simulink subsystem "BMS"  (R2024b)
settings: Solver=VariableStepAuto  StartTime=0.0  StopTime=10.0  RelTol=1e-3
undefined symbols (not defined in the file): Ambient, battery_builder_rtmsupport, ChargeKp, ChargerCC_A, ChargerKi, CoolantTemp, CurrOffset, gcbh, MaxChrgCurLim, MaxDchrgCurLim, MaxThLmt, MaxVoltLmt, MinThLmt, MinVoltLmt, Np, VoltOffset
libraries: nesl_utility x27, Batteries_lib x20, fl_lib x11, BatteryThermalManagement x1, BatteryCurrentManagement x1, BatteryBalancing x1
(part 2 of 4)

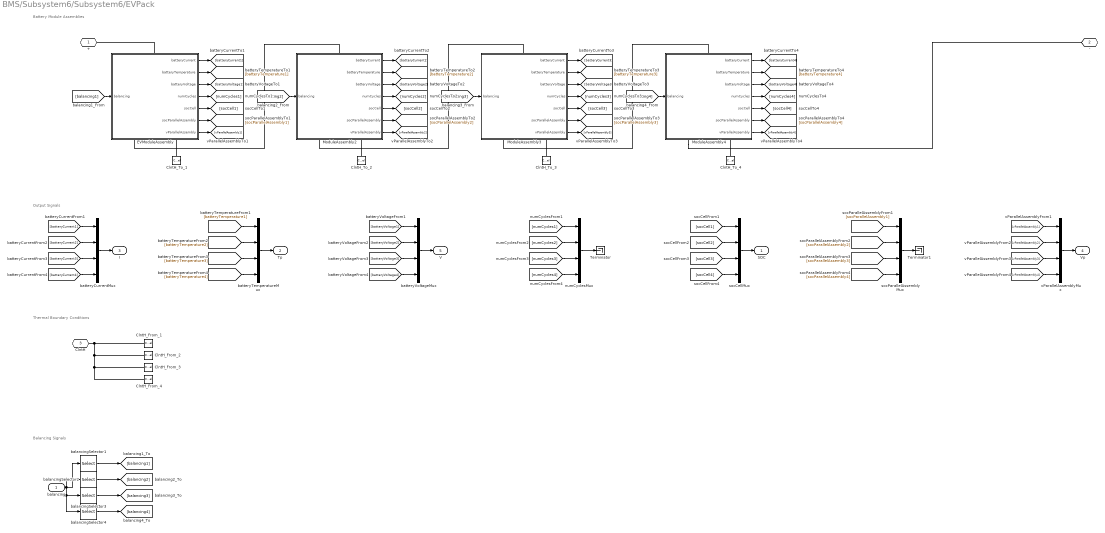
== system BMS/Subsystem6/Subsystem6/EVPack ==
  note: Balancing Signals
  note: Thermal Boundary Conditions
  note: Output Signals
  note: Battery Module Assemblies
  balancing : Inport  PortDimensions=100
  ClntH_From_1 : ConnectionLabel  Label=clntH_1
  ClntH_From_2 : ConnectionLabel  Label=clntH_2
  ClntH_From_3 : ConnectionLabel  Label=clntH_3
  ClntH_From_4 : ConnectionLabel  Label=clntH_4
  ClntH_To_1 : ConnectionLabel  Label=clntH_1
  ClntH_To_2 : ConnectionLabel  Label=clntH_2
  ClntH_To_3 : ConnectionLabel  Label=clntH_3
  ClntH_To_4 : ConnectionLabel  Label=clntH_4
  EVModuleAssembly : Subsystem  LoadFcn=battery_builder_rtmsupport('loadfcn',gcbh);
      settings: CopyFcn=battery_builder_rtmsupport('copyfcn',gcbh);  PreCopyFcn=battery_builder_rtmsupport('precopyfcn',gcbh);  PreDeleteFcn=battery_builder_rtmsupport('predeletefcn',gcbh);  PortSchema="{\"entries\":[{\"content\":{\"sides\":[{\"content\":{\"connectorIds\":[\"LConn1\"]},\"type\":\"ConnectorPlacement.EquallySpacedRectSide\",\"uuid\":\"3fa46d70-8935-4e0c-abb4-9c9b0d92b81b\"},{\"content\":{\"connectorIds\":[\"RConn1\",\"RConn2\"],\"side\":\"RIGHT\"},\"type\":\"ConnectorPlacement.EquallySpacedRectSide\",\"uuid\":\"6c8ace96-c3fc-41f9-a773-88712ff4ff02\"},{\"content\":{\"connectorIds\":[\"In1\"],\"side\":\"TOP\"},\"type\":\"ConnectorPlacement.EquallySpacedRectSide\",\"uuid\":\"16b2d02e-c4ca-4b99-b91f-f3cca8ade205\"},{\"content\":{\"connectorIds\":[\"Out1\",\"Out2\",\"Out3\",\"Out4\",\"Out5\",\"Out6\",\"Out7\"],\"side\":\"BOTTOM\"},\"type\":\"ConnectorPlacement.EquallySpacedRectSide\",\"uuid\":\"90084359-4b5d-48c4-95f3-9d483f7e7445\"}]},\"type\":\"ConnectorPlacement.EquallySpacedConnector\",\"uuid\":\"91dc49f4-abd8-4582-9e7e-23b88d2919e3\"}],\"packageUris\":[\"http://schema.mathworks.com/mf0/Connector/R2020b\"],\"version\":\"1.0\"}"
      mask Display: image('$imagefile')
  ModuleAssembly2 : Subsystem  LoadFcn=battery_builder_rtmsupport('loadfcn',gcbh);
      settings: CopyFcn=battery_builder_rtmsupport('copyfcn',gcbh);  PreCopyFcn=battery_builder_rtmsupport('precopyfcn',gcbh);  PreDeleteFcn=battery_builder_rtmsupport('predeletefcn',gcbh);  PortSchema="{\"entries\":[{\"content\":{\"sides\":[{\"content\":{\"connectorIds\":[\"LConn1\"]},\"type\":\"ConnectorPlacement.EquallySpacedRectSide\",\"uuid\":\"3fa46d70-8935-4e0c-abb4-9c9b0d92b81b\"},{\"content\":{\"connectorIds\":[\"RConn1\",\"RConn2\"],\"side\":\"RIGHT\"},\"type\":\"ConnectorPlacement.EquallySpacedRectSide\",\"uuid\":\"6c8ace96-c3fc-41f9-a773-88712ff4ff02\"},{\"content\":{\"connectorIds\":[\"In1\"],\"side\":\"TOP\"},\"type\":\"ConnectorPlacement.EquallySpacedRectSide\",\"uuid\":\"16b2d02e-c4ca-4b99-b91f-f3cca8ade205\"},{\"content\":{\"connectorIds\":[\"Out1\",\"Out2\",\"Out3\",\"Out4\",\"Out5\",\"Out6\",\"Out7\"],\"side\":\"BOTTOM\"},\"type\":\"ConnectorPlacement.EquallySpacedRectSide\",\"uuid\":\"90084359-4b5d-48c4-95f3-9d483f7e7445\"}]},\"type\":\"ConnectorPlacement.EquallySpacedConnector\",\"uuid\":\"91dc49f4-abd8-4582-9e7e-23b88d2919e3\"}],\"packageUris\":[\"http://schema.mathworks.com/mf0/Connector/R2020b\"],\"version\":\"1.0\"}"
      mask Display: image('$imagefile')
  ModuleAssembly3 : Subsystem  LoadFcn=battery_builder_rtmsupport('loadfcn',gcbh);
      settings: CopyFcn=battery_builder_rtmsupport('copyfcn',gcbh);  PreCopyFcn=battery_builder_rtmsupport('precopyfcn',gcbh);  PreDeleteFcn=battery_builder_rtmsupport('predeletefcn',gcbh);  PortSchema="{\"entries\":[{\"content\":{\"sides\":[{\"content\":{\"connectorIds\":[\"LConn1\"]},\"type\":\"ConnectorPlacement.EquallySpacedRectSide\",\"uuid\":\"3fa46d70-8935-4e0c-abb4-9c9b0d92b81b\"},{\"content\":{\"connectorIds\":[\"RConn1\",\"RConn2\"],\"side\":\"RIGHT\"},\"type\":\"ConnectorPlacement.EquallySpacedRectSide\",\"uuid\":\"6c8ace96-c3fc-41f9-a773-88712ff4ff02\"},{\"content\":{\"connectorIds\":[\"In1\"],\"side\":\"TOP\"},\"type\":\"ConnectorPlacement.EquallySpacedRectSide\",\"uuid\":\"16b2d02e-c4ca-4b99-b91f-f3cca8ade205\"},{\"content\":{\"connectorIds\":[\"Out1\",\"Out2\",\"Out3\",\"Out4\",\"Out5\",\"Out6\",\"Out7\"],\"side\":\"BOTTOM\"},\"type\":\"ConnectorPlacement.EquallySpacedRectSide\",\"uuid\":\"90084359-4b5d-48c4-95f3-9d483f7e7445\"}]},\"type\":\"ConnectorPlacement.EquallySpacedConnector\",\"uuid\":\"91dc49f4-abd8-4582-9e7e-23b88d2919e3\"}],\"packageUris\":[\"http://schema.mathworks.com/mf0/Connector/R2020b\"],\"version\":\"1.0\"}"
      mask Display: image('$imagefile')
  ModuleAssembly4 : Subsystem  LoadFcn=battery_builder_rtmsupport('loadfcn',gcbh);
      settings: CopyFcn=battery_builder_rtmsupport('copyfcn',gcbh);  PreCopyFcn=battery_builder_rtmsupport('precopyfcn',gcbh);  PreDeleteFcn=battery_builder_rtmsupport('predeletefcn',gcbh);  PortSchema="{\"entries\":[{\"content\":{\"sides\":[{\"content\":{\"connectorIds\":[\"LConn1\"]},\"type\":\"ConnectorPlacement.EquallySpacedRectSide\",\"uuid\":\"3fa46d70-8935-4e0c-abb4-9c9b0d92b81b\"},{\"content\":{\"connectorIds\":[\"RConn1\",\"RConn2\"],\"side\":\"RIGHT\"},\"type\":\"ConnectorPlacement.EquallySpacedRectSide\",\"uuid\":\"6c8ace96-c3fc-41f9-a773-88712ff4ff02\"},{\"content\":{\"connectorIds\":[\"In1\"],\"side\":\"TOP\"},\"type\":\"ConnectorPlacement.EquallySpacedRectSide\",\"uuid\":\"16b2d02e-c4ca-4b99-b91f-f3cca8ade205\"},{\"content\":{\"connectorIds\":[\"Out1\",\"Out2\",\"Out3\",\"Out4\",\"Out5\",\"Out6\",\"Out7\"],\"side\":\"BOTTOM\"},\"type\":\"ConnectorPlacement.EquallySpacedRectSide\",\"uuid\":\"90084359-4b5d-48c4-95f3-9d483f7e7445\"}]},\"type\":\"ConnectorPlacement.EquallySpacedConnector\",\"uuid\":\"91dc49f4-abd8-4582-9e7e-23b88d2919e3\"}],\"packageUris\":[\"http://schema.mathworks.com/mf0/Connector/R2020b\"],\"version\":\"1.0\"}"
      mask Display: image('$imagefile')
  Terminator : Terminator
  Terminator1 : Terminator
  balancingSelector1 : Selector  InputPortWidth=100  IndexOptions=Index vector (dialog)  Indices="[1   2   3   4   5   6   7   8   9  10  11  12  13  14  15  16  17  18  19  20  21  22  23  24  25]"  OutputSizes=1
  balancingSelector2 : Selector  InputPortWidth=100  IndexOptions=Index vector (dialog)  Indices="[26  27  28  29  30  31  32  33  34  35  36  37  38  39  40  41  42  43  44  45  46  47  48  49  50]"  OutputSizes=1
  balancingSelector3 : Selector  InputPortWidth=100  IndexOptions=Index vector (dialog)  Indices="[51  52  53  54  55  56  57  58  59  60  61  62  63  64  65  66  67  68  69  70  71  72  73  74  75]"  OutputSizes=1
  balancingSelector4 : Selector  InputPortWidth=100  IndexOptions=Index vector (dialog)  Indices="[76   77   78   79   80   81   82   83   84   85   86   87   88   89   90   91   92   93   94   95   96   97   98   99  100]"  OutputSizes=1
  batteryCurrentMux : Mux
  batteryTemperatureMux : Mux
  batteryVoltageMux : Mux
  numCyclesMux : Mux
  socCellMux : Mux
  socParallelAssemblyMux : Mux
  vParallelAssemblyMux : Mux
  + : PMIOPort  Side=Left
  - : PMIOPort  Port=2  Side=Right
  ClntH : PMIOPort  Port=3  Side=Right  ConnectionType=Connection: foundation.thermal.thermal
  SOC : Outport
  Tp : Outport  Port=2
  I : Outport  Port=3
  Vp : Outport  Port=4
  V : Outport  Port=5
  wires:
  balancingSelector4/1 -> [balancing4]
  [balancing4] -> ModuleAssembly4/1(balancing)
  balancingSelector3/1 -> [balancing3]
  [balancing3] -> ModuleAssembly3/1(balancing)
  balancingSelector2/1 -> [balancing2]
  [balancing2] -> ModuleAssembly2/1(balancing)
  balancingSelector1/1 -> [balancing1]
  balancing/1 -> balancingSelector4/1, balancingSelector3/1, balancingSelector2/1, balancingSelector1/1
  [balancing1] -> EVModuleAssembly/1(balancing)
  [vParallelAssembly4] -> vParallelAssemblyMux/4
  ModuleAssembly4/7(vParallelAssembly) -> [vParallelAssembly4]
  [socParallelAssembly4] -> socParallelAssemblyMux/4
  ModuleAssembly4/6(socParallelAssembly) -> [socParallelAssembly4]
  [socCell4] -> socCellMux/4
  ModuleAssembly4/5(socCell) -> [socCell4]
  [numCycles4] -> numCyclesMux/4
  ModuleAssembly4/4(numCycles) -> [numCycles4]
  [batteryVoltage4] -> batteryVoltageMux/4
  ModuleAssembly4/3(batteryVoltage) -> [batteryVoltage4]
  [batteryTemperature4] -> batteryTemperatureMux/4
  ModuleAssembly4/2(batteryTemperature) -> [batteryTemperature4]
  [batteryCurrent4] -> batteryCurrentMux/4
  ModuleAssembly4/1(batteryCurrent) -> [batteryCurrent4]
  [vParallelAssembly3] -> vParallelAssemblyMux/3
  ModuleAssembly3/7(vParallelAssembly) -> [vParallelAssembly3]
  [socParallelAssembly3] -> socParallelAssemblyMux/3
  ModuleAssembly3/6(socParallelAssembly) -> [socParallelAssembly3]
  [socCell3] -> socCellMux/3
  ModuleAssembly3/5(socCell) -> [socCell3]
  [numCycles3] -> numCyclesMux/3
  ModuleAssembly3/4(numCycles) -> [numCycles3]
  [batteryVoltage3] -> batteryVoltageMux/3
  ModuleAssembly3/3(batteryVoltage) -> [batteryVoltage3]
  [batteryTemperature3] -> batteryTemperatureMux/3
  ModuleAssembly3/2(batteryTemperature) -> [batteryTemperature3]
  [batteryCurrent3] -> batteryCurrentMux/3
  ModuleAssembly3/1(batteryCurrent) -> [batteryCurrent3]
  [vParallelAssembly2] -> vParallelAssemblyMux/2
  ModuleAssembly2/7(vParallelAssembly) -> [vParallelAssembly2]
  [socParallelAssembly2] -> socParallelAssemblyMux/2
  ModuleAssembly2/6(socParallelAssembly) -> [socParallelAssembly2]
  [socCell2] -> socCellMux/2
  ModuleAssembly2/5(socCell) -> [socCell2]
  [numCycles2] -> numCyclesMux/2
  ModuleAssembly2/4(numCycles) -> [numCycles2]
  [batteryVoltage2] -> batteryVoltageMux/2
  ModuleAssembly2/3(batteryVoltage) -> [batteryVoltage2]
  [batteryTemperature2] -> batteryTemperatureMux/2
  ModuleAssembly2/2(batteryTemperature) -> [batteryTemperature2]
  [batteryCurrent2] -> batteryCurrentMux/2
  ModuleAssembly2/1(batteryCurrent) -> [batteryCurrent2]
  [vParallelAssembly1] -> vParallelAssemblyMux/1
  vParallelAssemblyMux/1 -> Vp/1
  EVModuleAssembly/7(vParallelAssembly) -> [vParallelAssembly1]
  [socParallelAssembly1] -> socParallelAssemblyMux/1
  socParallelAssemblyMux/1 -> Terminator1/1
  EVModuleAssembly/6(socParallelAssembly) -> [socParallelAssembly1]
  [socCell1] -> socCellMux/1
  socCellMux/1 -> SOC/1
  EVModuleAssembly/5(socCell) -> [socCell1]
  [numCycles1] -> numCyclesMux/1
  numCyclesMux/1 -> Terminator/1
  EVModuleAssembly/4(numCycles) -> [numCycles1]
  [batteryVoltage1] -> batteryVoltageMux/1
  batteryVoltageMux/1 -> V/1
  EVModuleAssembly/3(batteryVoltage) -> [batteryVoltage1]
  [batteryTemperature1] -> batteryTemperatureMux/1
  batteryTemperatureMux/1 -> Tp/1
  EVModuleAssembly/2(batteryTemperature) -> [batteryTemperature1]
  [batteryCurrent1] -> batteryCurrentMux/1
  batteryCurrentMux/1 -> I/1
  EVModuleAssembly/1(batteryCurrent) -> [batteryCurrent1]
  connections:
  ClntH_To_4/LConn1 -- ModuleAssembly4/RConn2
  ClntH_To_3/LConn1 -- ModuleAssembly3/RConn2
  ClntH_To_2/LConn1 -- ModuleAssembly2/RConn2
  ClntH_From_4/LConn1 -- ClntH/RConn1 -- ClntH_From_1/LConn1 -- ClntH_From_2/LConn1 -- ClntH_From_3/LConn1
  ClntH_To_1/LConn1 -- EVModuleAssembly/RConn2
  ModuleAssembly4/RConn1 -- -/RConn1
  EVModuleAssembly/LConn1 -- +/RConn1
  ModuleAssembly4/LConn1 -- ModuleAssembly3/RConn1
  ModuleAssembly3/LConn1 -- ModuleAssembly2/RConn1
  ModuleAssembly2/LConn1 -- EVModuleAssembly/RConn1

== system BMS/Subsystem6/BMS/Battery Protection Logic/State Flow ==
  Bus Element In11 : Inport  PortName=StateInput  Element=Current
  Bus Element In1 : Inport  PortName=StateInput  Element=CurLmt
  Bus Element In2 : Inport  PortName=StateInput  Element=Volt
  Bus Element In4 : Inport  PortName=StateInput  Element=Tp
  Bus Element In6 : Inport  PortName=StateInput  Element=BatSoC
  Bus Element In7 : Inport  PortName=StateInput  Element=BatCmd
  Bus Element In8 : Inport  PortName=StateInput  Element=FaultReset
  Bus Creator8 : BusCreator  Inputs=5
  Bus Creator9 : BusCreator  Inputs=4
  Delay{,1..3} (4 alike) : Delay  DelayLength=1
  Fault Protection : Stateflow chart  TreatAsAtomicUnit=on
      settings: PortSchema="{\"entries\":[{\"content\":{\"sides\":[{\"content\":{\"connectorIds\":[\"In1\",\"In2\",\"In3\",\"In4\",\"In5\",\"In6\",\"In7\"]},\"type\":\"ConnectorPlacement.EquallySpacedRectSide\",\"uuid\":\"7222f55a-2aef-4ca8-adbd-e86ed030f82f\"},{\"content\":{\"connectorIds\":[\"Out5\",\"Out6\",\"Out10\",\"Out9\",\"Out4\",\"Out1\",\"Out2\",\"Out3\",\"Out7\",\"Out8\"],\"side\":\"RIGHT\"},\"type\":\"ConnectorPlacement.EquallySpacedRectSide\",\"uuid\":\"bfa2f4e3-3563-4466-8725-57bf2336ec66\"},{\"content\":{\"connectorIds\":[],\"side\":\"TOP\"},\"type\":\"ConnectorPlacement.EquallySpacedRectSide\",\"uuid\":\"7b1e9a44-7135-4c45-bb2b-0152be29b46d\"}]},\"type\":\"ConnectorPlacement.EquallySpacedConnector\",\"uuid\":\"80032a24-3823-40c6-b797-ffbc29f7d345\"}],\"packageUris\":[\"http://schema.mathworks.com/mf0/Connector/R2020b\"],\"version\":\"1.0\"}"
  Out Bus Element : Outport  PortName=StateOut  Element=RelayRq
  Out Bus Element1 : Outport  PortName=StateOut  Element=BatSt
  Out Bus Element2 : Outport  PortName=StateOut  Element=Fault
  wires:
  Bus Element In7/1 -> Fault Protection/6(BatCmd)
  Bus Element In8/1 -> Fault Protection/7(FaultReset)
  Bus Element In2/1 -> Fault Protection/3(Volt)
  Bus Element In1/1 -> Fault Protection/2(CurLmt)
  Bus Element In11/1 -> Fault Protection/1(I)
  Bus Element In4/1 -> Fault Protection/4(Tp)
  Bus Element In6/1 -> Fault Protection/5(BatSoC)
  Bus Creator9/1 -> Out Bus Element/1  "RelayRq"
  Bus Creator8/1 -> Out Bus Element2/1  "Fault"
  Fault Protection/5(Rpos) -> Delay/1  "RelayPos"
  Fault Protection/6(Rneg) -> Delay1/1  "RelayNeg"
  Fault Protection/10(RelDchg) -> Delay2/1  "RelayDchg"
  Fault Protection/9(RelChg) -> Delay3/1  "RelayChg"
  Fault Protection/4(BatSt) -> Out Bus Element1/1  "BatSt"
  Fault Protection/2(FaultElec) -> Bus Creator8/2  "FaultElec"
  Fault Protection/3(FaultTh) -> Bus Creator8/3  "FaultTh"
  Fault Protection/7(FaultVolt) -> Bus Creator8/4  "FaultVolt"
  Fault Protection/8(FaultDisp) -> Bus Creator8/5  "FaultDisp"
  Fault Protection/1(FaultDet) -> Bus Creator8/1  "FaultDet"
  Delay/1 -> Bus Creator9/1  "RelayPos"
  Delay1/1 -> Bus Creator9/2  "RelayNeg"
  Delay2/1 -> Bus Creator9/3  "RelayDchg"
  Delay3/1 -> Bus Creator9/4  "RelayChg"

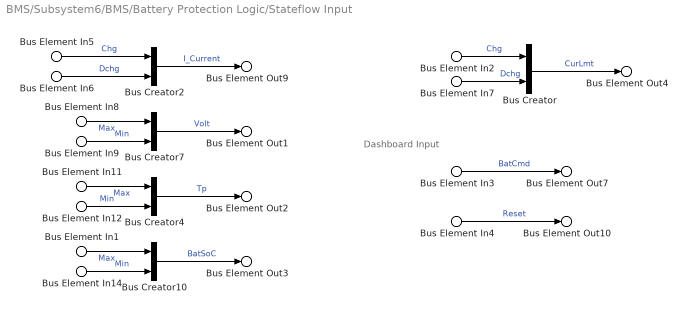
== system BMS/Subsystem6/BMS/Battery Protection Logic/Stateflow Input ==
  note: Dashboard Input
  Bus Element In1 : Inport  PortName=SoC  Element=CellSoCmax
  Bus Element In14 : Inport  PortName=SoC  Element=CellSoCmin
  Bus Element In2 : Inport  Port=2  PortName=Current  Element=CurChgLmt
  Bus Element In7 : Inport  Port=2  PortName=Current  Element=CurDchLmt
  Bus Element In5 : Inport  Port=2  PortName=Current  Element=CurChgDchg.Chg
  Bus Element In6 : Inport  Port=2  PortName=Current  Element=CurChgDchg.Dchg
  Bus Element In8 : Inport  Port=3  PortName=Sensor  Element=CellVoltMax
  Bus Element In9 : Inport  Port=3  PortName=Sensor  Element=CellVoltMin
  Bus Element In11 : Inport  Port=3  PortName=Sensor  Element=CellTempMax
  Bus Element In12 : Inport  Port=3  PortName=Sensor  Element=CellTempMin
  Bus Element In3 : Inport  Port=3  PortName=Sensor  Element=BatCmd
  Bus Element In4 : Inport  Port=3  PortName=Sensor  Element=Reset
  Bus Creator : BusCreator  Inputs=2  OutDataTypeStr=Bus: I_Current
  Bus Creator10 : BusCreator  Inputs=2  OutDataTypeStr=Bus: MaxMinLimit
  Bus Creator2 : BusCreator  Inputs=2  OutDataTypeStr=Bus: I_Current
  Bus Creator4 : BusCreator  Inputs=2  OutDataTypeStr=Bus: MaxMinLimit
  Bus Creator7 : BusCreator  Inputs=2  OutDataTypeStr=Bus: CellVoltage  NonVirtualBus=on
  Bus Element Out9 : Outport  PortName=StateInput  Element=Current
  Bus Element Out1 : Outport  PortName=StateInput  Element=Volt
  Bus Element Out2 : Outport  PortName=StateInput  Element=Tp
  Bus Element Out3 : Outport  PortName=StateInput  Element=BatSoC
  Bus Element Out4 : Outport  PortName=StateInput  Element=CurLmt
  Bus Element Out7 : Outport  PortName=StateInput  Element=BatCmd
  Bus Element Out10 : Outport  PortName=StateInput  Element=FaultReset
  wires:
  Bus Element In7/1 -> Bus Creator/2  "Dchg"
  Bus Element In2/1 -> Bus Creator/1  "Chg"
  Bus Creator7/1 -> Bus Element Out1/1  "Volt"
  Bus Creator2/1 -> Bus Element Out9/1  "I_Current"
  Bus Creator4/1 -> Bus Element Out2/1  "Tp"
  Bus Element In3/1 -> Bus Element Out7/1  "BatCmd"
  Bus Element In4/1 -> Bus Element Out10/1  "Reset"
  Bus Element In14/1 -> Bus Creator10/2  "Min"
  Bus Element In1/1 -> Bus Creator10/1  "Max"
  Bus Element In6/1 -> Bus Creator2/2  "Dchg"
  Bus Element In5/1 -> Bus Creator2/1  "Chg"
  Bus Creator10/1 -> Bus Element Out3/1  "BatSoC"
  Bus Element In11/1 -> Bus Creator4/1  "Max"
  Bus Creator/1 -> Bus Element Out4/1  "CurLmt"
  Bus Element In9/1 -> Bus Creator7/2  "Min"
  Bus Element In8/1 -> Bus Creator7/1  "Max"
  Bus Element In12/1 -> Bus Creator4/2  "Min"

== system BMS/Subsystem6/BMS/MinMax Current Limiter/Current Directional ==
  CurDir : Inport
  Cur : Inport  Port=2
  Abs : Abs  SaturateOnIntegerOverflow=off
  Bus Creator2 : BusCreator  Inputs=2  OutDataTypeStr=Bus: I_Current
  Bus Selector : BusSelector  OutputSignals=Chg,Dsch
  Gain : Gain  Gain=-1
  Product : Product
  Product1 : Product
  I_Current : Outport
  wires:
  Product1/1 -> Bus Creator2/2  "Dchg"
  Bus Creator2/1 -> I_Current/1  "I_Current"
  Product/1 -> Bus Creator2/1  "Chg"
  Bus Selector/2 -> Product1/1  "<Dsch>"
  Bus Selector/1 -> Gain/1  "<Chg>"
  CurDir/1 -> Bus Selector/1
  Abs/1 -> Product1/2, Product/2
  Cur/1 -> Abs/1
  Gain/1 -> Product/1

== system BMS/Subsystem6/BMS/MinMax Current Limiter/OCprotection ==
  Cur : Inport
  VoltMax : Inport  Port=2
  CellTpMax : Inport  Port=3
  CellTpMin : Inport  Port=4
  Add : Sum  Inputs=-+
  ChrgCurrLimitMaxTp : Lookup_n-D  NumberOfTableDimensions=1  BreakpointsForDimension1="single([313  318  323  340 350])"  BreakpointsForDimension3=[5, 7]  Table=single([1.0 0.8 0.5 0.3 0])  ExtrapMethod=Clip  UseLastTableValue=on  InternalRulePriority=Speed  RndMeth=Simplest
  ChrgCurrLimitMinTp : Lookup_n-D  NumberOfTableDimensions=1  BreakpointsForDimension1=single([258 263 268 273 278 283 288])  BreakpointsForDimension3=[5, 7]  Table="single([0.1 0.2  0.3 0.3 0.5 1.0 1.0])"  ExtrapMethod=Clip  UseLastTableValue=on  InternalRulePriority=Speed  RndMeth=Simplest
  ChrgCurrLimitVolt : Lookup_n-D  NumberOfTableDimensions=1  BreakpointsForDimension1=single([3.9 4.0 4.15 4.2])  BreakpointsForDimension3=[5, 7]  Table="single([1.0 0.8 0.3  0.3])"  ExtrapMethod=Clip  UseLastTableValue=on  InternalRulePriority=Speed  RndMeth=Simplest
  Constant : Constant  Value=10
  MaxChrgCurLim : Gain  Gain=-MaxChrgCurLim
  Min : MinMax  Inputs=3
  Np_Module : Gain  Gain=Np
  Relational Operator : RelationalOperator  Operator=<=  OutDataTypeStr=boolean  RndMeth=Simplest  InputSameDT=off
  Scope : Scope
  OCWarn : Outport
  ChrgCurLim : Outport  Port=2
  wires:
  Relational Operator/1 -> OCWarn/1
  [ChrgCurLim] -> Add/2
  Cur/1 -> Relational Operator/2
  Min/1 -> MaxChrgCurLim/1
  ChrgCurrLimitMinTp/1 -> Min/3  "MinTpChrgCurrLim"
  ChrgCurrLimitMaxTp/1 -> Min/2  "MaxTpChrgCurrLim"
  CellTpMin/1 -> ChrgCurrLimitMinTp/1
  CellTpMax/1 -> ChrgCurrLimitMaxTp/1
  Np_Module/1 -> Scope/1, [ChrgCurLim], ChrgCurLim/1  "CurChrgLmt"
  MaxChrgCurLim/1 -> Np_Module/1
  ChrgCurrLimitVolt/1 -> Min/1  "ChrgCurrLimVolt"
  VoltMax/1 -> ChrgCurrLimitVolt/1
  Constant/1 -> Add/1
  Add/1 -> Relational Operator/1

== system BMS/Subsystem6/BMS/MinMax Current Limiter/ODprotection ==
  Cur : Inport
  VoltMin : Inport  Port=2
  CellTpMax : Inport  Port=3
  CellTpMin : Inport  Port=4
  Add : Sum  Inputs=-+
  Constant : Constant  Value=10
  DchrgCurLim : Gain  Gain=MaxDchrgCurLim
  DischCurrLimitMaxTp : Lookup_n-D  NumberOfTableDimensions=1  BreakpointsForDimension1=single([313, 318, 323, 333, 350])  BreakpointsForDimension3=[5, 7]  Table=single([1,0.7, 0.5, 0.3, 0])  ExtrapMethod=Clip  UseLastTableValue=on  InternalRulePriority=Speed  RndMeth=Simplest
  DischCurrLimitMinTp : Lookup_n-D  NumberOfTableDimensions=1  BreakpointsForDimension1="single([263, 268,    273,   278, 283, 288, 293])"  BreakpointsForDimension3=[5, 7]  Table="single([0,  0.2, 0.3, 0.5, 0.75, 1, 1])"  ExtrapMethod=Clip  UseLastTableValue=on  InternalRulePriority=Speed  RndMeth=Simplest
  DischCurrLimitVolt : Lookup_n-D  NumberOfTableDimensions=1  BreakpointsForDimension1=single([2.5;3;3.5;4.2])  BreakpointsForDimension3=[5, 7]  Table=single([0 0.25 0.5 0.75])  ExtrapMethod=Clip  UseLastTableValue=on  InternalRulePriority=Speed  RndMeth=Simplest
  Min : MinMax  Inputs=3
  Np_Module : Gain  Gain=Np
  Relational Operator : RelationalOperator  Operator=<=  OutDataTypeStr=boolean  RndMeth=Simplest  InputSameDT=off
  DschCurLim : Outport
  ODWarn : Outport  Port=2
  wires:
  VoltMin/1 -> DischCurrLimitVolt/1
  DischCurrLimitVolt/1 -> Min/1  "DischCurrLimVolt"
  DchrgCurLim/1 -> Np_Module/1
  Np_Module/1 -> DschCurLim/1, [DschCurLim]  "CurDchLmt"
  CellTpMax/1 -> DischCurrLimitMaxTp/1
  CellTpMin/1 -> DischCurrLimitMinTp/1
  DischCurrLimitMaxTp/1 -> Min/2  "DischCurrLimMaxTp"
  DischCurrLimitMinTp/1 -> Min/3  "DischCurrLimMinTp"
  Min/1 -> DchrgCurLim/1
  Cur/1 -> Relational Operator/2
  [DschCurLim] -> Add/2
  Relational Operator/1 -> ODWarn/1
  Add/1 -> Relational Operator/1
  Constant/1 -> Add/1

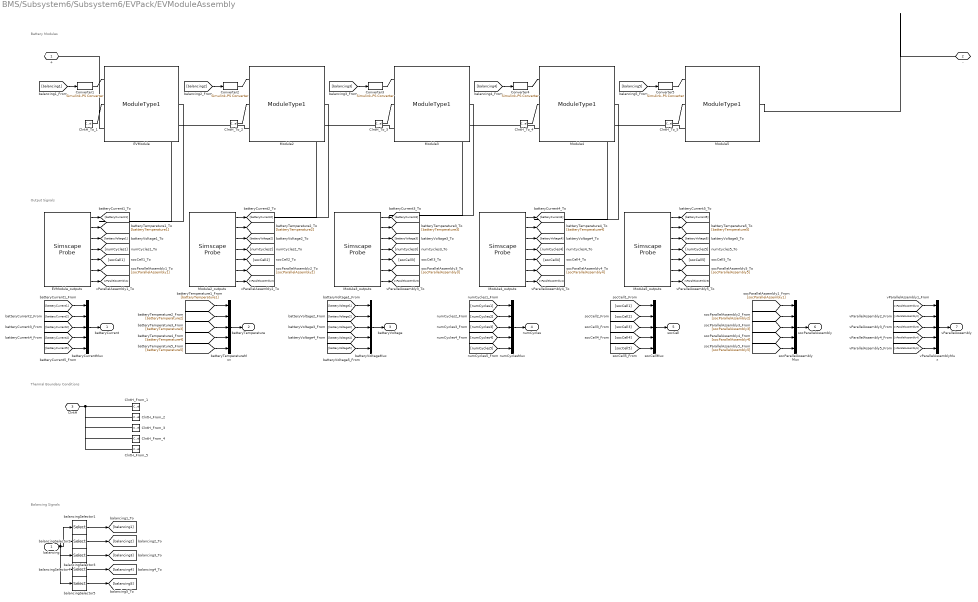
== system BMS/Subsystem6/Subsystem6/EVPack/EVModuleAssembly ==
  note: Battery Modules
  note: Output Signals
  note: Thermal Boundary Conditions
  note: Balancing Signals
  balancing : Inport  PortDimensions=25
  ClntH_From_1 : ConnectionLabel  Label=clntH_1
  ClntH_From_2 : ConnectionLabel  Label=clntH_2
  ClntH_From_3 : ConnectionLabel  Label=clntH_3
  ClntH_From_4 : ConnectionLabel  Label=clntH_4
  ClntH_From_5 : ConnectionLabel  Label=clntH_5
  ClntH_To_1 : ConnectionLabel  Label=clntH_1
  ClntH_To_2 : ConnectionLabel  Label=clntH_2
  ClntH_To_3 : ConnectionLabel  Label=clntH_3
  ClntH_To_4 : ConnectionLabel  Label=clntH_4
  ClntH_To_5 : ConnectionLabel  Label=clntH_5
  Converter{1..5} (5 alike) : nesl_utility/Simulink-PS Converter  PhysicalDomain=network_engine_domain  SubClassName=ps_input  LeftPortType=input  RightPortType=output  PseudoPeriodic=off  Frequencies=[]  NoiseDistribution=none  NoiseParameters=[]  Unit=1  AffineConversion=off  FilteringAndDerivatives=provide  SimscapeFilterOrder=1  InputFilterTimeConstant=0.001  UdotUserProvided=0
  EVModule : Batteries_lib/Modules/ModuleType1  BatteryCapacityCell=27 A*hr  ExtrapolationMethodCell=simscape.enum.extrapolation.nearest  SOCBreakpointsCell=[0, .1, .25, .5, .75, .9, 1]  TemperatureBreakpointsCell=[278, 293, 313] K  OpenCircuitVoltageThermalCell=[3.49, 3.5, 3.51; 3.55, 3.57, 3.56; 3.62, 3.63, 3.64; 3.71, 3.71, 3.72; 3.91, 3.93, 3.94; 4.07, 4.08, 4.08; 4.19, 4.19, 4.19] V  VoltageRangeCell=[0, inf] V  ResistanceSOCBreakpointsCell=[0, .1, .25, .5, .75, .9, 1]  ResistanceTemperatureBreakpointsCell=[278, 293, 313] K  R0ThermalCell=[.0117, .0085, .009; .011, .0085, .009; .0114, .0087, .0092; .0107, .0082, .0088; .0107, .0083, .0091; .0113, .0085, .0089; .0116, .0085, .0089] Ohm  BatteryThermalMassCell=100 J/K  CoolantResistance=1.2 K/W  CellBalancingClosedResistance=0.01 Ohm  CellBalancingOpenConductance=1e-8 1/Ohm  CellBalancingThreshold=0.5  CellBalancingResistance=50 Ohm  P=4  S=5  socCell_specify=off  socCell_priority=High  socCell=1  socCell_nominal_specify=off  socCell_nominal_value=1  socCell_nominal_unit=1  numCycles_specify=off  numCycles_priority=High  numCycles=0  numCycles_nominal_specify=off  numCycles_nominal_value=1  numCycles_nominal_unit=1  batteryVoltage_specify=off  batteryVoltage_priority=None  batteryVoltage=0 V  batteryVoltage_nominal_specify=off  batteryVoltage_nominal_value=1  batteryVoltage_nominal_unit=V  batteryCurrent_specify=off  batteryCurrent_priority=None  batteryCurrent=0 A  batteryCurrent_nominal_specify=off  batteryCurrent_nominal_value=1  batteryCurrent_nominal_unit=A  batteryTemperature_specify=off  batteryTemperature_priority=High  batteryTemperature=298.15 K  batteryTemperature_nominal_specify=off  batteryTemperature_nominal_value=1  batteryTemperature_nominal_unit=K  vParallelAssembly_specify=off  vParallelAssembly_priority=None  vParallelAssembly=repmat(0, 5, 1) V  vParallelAssembly_nominal_specify=off  vParallelAssembly_nominal_value=1  vParallelAssembly_nominal_unit=V  socParallelAssembly_specify=off  socParallelAssembly_priority=None  socParallelAssembly=repmat(1, 5, 1)  socParallelAssembly_nominal_specify=off  socParallelAssembly_nominal_value=1  socParallelAssembly_nominal_unit=1
      settings: InternalSimscapePortConfiguration="{\"Bottom\":[{\"id\":\"n\",\"label\":\"-\",\"type\":\"foundation.electrical.electrical\"}],\"Left\":[{\"id\":\"enableCellBalancing\",\"label\":\"CB\",\"type\":\"input\"},{\"id\":\"ClntH\",\"label\":\"ClntH\",\"type\":\"foundation.thermal.thermal\"}],\"Right\":[],\"Top\":[{\"id\":\"p\",\"label\":\"+\",\"type\":\"foundation.electrical.electrical\"}]}"
  EVModule_outputs : SimscapeProbe  BoundBlock=1450  Variables="{\"batteryCurrent\":{\"Unit\":\"A\",\"PortLabel\":\"batteryCurrent\",\"Probing\":\"ON\"},\"batteryTemperature\":{\"Unit\":\"K\",\"PortLabel\":\"batteryTemperature\",\"Probing\":\"ON\"},\"batteryVoltage\":{\"Unit\":\"V\",\"PortLabel\":\"batteryVoltage\",\"Probing\":\"ON\"},\"numCycles\":{\"Unit\":\"1\",\"PortLabel\":\"numCycles\",\"Probing\":\"ON\"},\"socCell\":{\"Unit\":\"1\",\"PortLabel\":\"socCell\",\"Probing\":\"ON\"},\"socParallelAssembly\":{\"Unit\":\"1\",\"PortLabel\":\"socParallelAssembly\",\"Probing\":\"ON\"},\"vParallelAssembly\":{\"Unit\":\"V\",\"PortLabel\":\"vParallelAssembly\",\"Probing\":\"ON\"}}"
  Module{2..5} (4 alike) : Batteries_lib/Modules/ModuleType1  BatteryCapacityCell=27 A*hr  ExtrapolationMethodCell=simscape.enum.extrapolation.nearest  SOCBreakpointsCell=[0, .1, .25, .5, .75, .9, 1]  TemperatureBreakpointsCell=[278, 293, 313] K  OpenCircuitVoltageThermalCell=[3.49, 3.5, 3.51; 3.55, 3.57, 3.56; 3.62, 3.63, 3.64; 3.71, 3.71, 3.72; 3.91, 3.93, 3.94; 4.07, 4.08, 4.08; 4.19, 4.19, 4.19] V  VoltageRangeCell=[0, inf] V  ResistanceSOCBreakpointsCell=[0, .1, .25, .5, .75, .9, 1]  ResistanceTemperatureBreakpointsCell=[278, 293, 313] K  R0ThermalCell=[.0117, .0085, .009; .011, .0085, .009; .0114, .0087, .0092; .0107, .0082, .0088; .0107, .0083, .0091; .0113, .0085, .0089; .0116, .0085, .0089] Ohm  BatteryThermalMassCell=100 J/K  CoolantResistance=1.2 K/W  CellBalancingClosedResistance=0.01 Ohm  CellBalancingOpenConductance=1e-8 1/Ohm  CellBalancingThreshold=0.5  CellBalancingResistance=50 Ohm  P=4  S=5  socCell_specify=off  socCell_priority=High  socCell=1  socCell_nominal_specify=off  socCell_nominal_value=1  socCell_nominal_unit=1  numCycles_specify=off  numCycles_priority=High  numCycles=0  numCycles_nominal_specify=off  numCycles_nominal_value=1  numCycles_nominal_unit=1  batteryVoltage_specify=off  batteryVoltage_priority=None  batteryVoltage=0 V  batteryVoltage_nominal_specify=off  batteryVoltage_nominal_value=1  batteryVoltage_nominal_unit=V  batteryCurrent_specify=off  batteryCurrent_priority=None  batteryCurrent=0 A  batteryCurrent_nominal_specify=off  batteryCurrent_nominal_value=1  batteryCurrent_nominal_unit=A  batteryTemperature_specify=off  batteryTemperature_priority=High  batteryTemperature=298.15 K  batteryTemperature_nominal_specify=off  batteryTemperature_nominal_value=1  batteryTemperature_nominal_unit=K  vParallelAssembly_specify=off  vParallelAssembly_priority=None  vParallelAssembly=repmat(0, 5, 1) V  vParallelAssembly_nominal_specify=off  vParallelAssembly_nominal_value=1  vParallelAssembly_nominal_unit=V  socParallelAssembly_specify=off  socParallelAssembly_priority=None  socParallelAssembly=repmat(1, 5, 1)  socParallelAssembly_nominal_specify=off  socParallelAssembly_nominal_value=1  socParallelAssembly_nominal_unit=1
      settings: InternalSimscapePortConfiguration="{\"Bottom\":[{\"id\":\"n\",\"label\":\"-\",\"type\":\"foundation.electrical.electrical\"}],\"Left\":[{\"id\":\"enableCellBalancing\",\"label\":\"CB\",\"type\":\"input\"},{\"id\":\"ClntH\",\"label\":\"ClntH\",\"type\":\"foundation.thermal.thermal\"}],\"Right\":[],\"Top\":[{\"id\":\"p\",\"label\":\"+\",\"type\":\"foundation.electrical.electrical\"}]}"
  Module2_outputs : SimscapeProbe  BoundBlock=1452  Variables="{\"batteryCurrent\":{\"Unit\":\"A\",\"PortLabel\":\"batteryCurrent\",\"Probing\":\"ON\"},\"batteryTemperature\":{\"Unit\":\"K\",\"PortLabel\":\"batteryTemperature\",\"Probing\":\"ON\"},\"batteryVoltage\":{\"Unit\":\"V\",\"PortLabel\":\"batteryVoltage\",\"Probing\":\"ON\"},\"numCycles\":{\"Unit\":\"1\",\"PortLabel\":\"numCycles\",\"Probing\":\"ON\"},\"socCell\":{\"Unit\":\"1\",\"PortLabel\":\"socCell\",\"Probing\":\"ON\"},\"socParallelAssembly\":{\"Unit\":\"1\",\"PortLabel\":\"socParallelAssembly\",\"Probing\":\"ON\"},\"vParallelAssembly\":{\"Unit\":\"V\",\"PortLabel\":\"vParallelAssembly\",\"Probing\":\"ON\"}}"
  Module3_outputs : SimscapeProbe  BoundBlock=1454  Variables="{\"batteryCurrent\":{\"Unit\":\"A\",\"PortLabel\":\"batteryCurrent\",\"Probing\":\"ON\"},\"batteryTemperature\":{\"Unit\":\"K\",\"PortLabel\":\"batteryTemperature\",\"Probing\":\"ON\"},\"batteryVoltage\":{\"Unit\":\"V\",\"PortLabel\":\"batteryVoltage\",\"Probing\":\"ON\"},\"numCycles\":{\"Unit\":\"1\",\"PortLabel\":\"numCycles\",\"Probing\":\"ON\"},\"socCell\":{\"Unit\":\"1\",\"PortLabel\":\"socCell\",\"Probing\":\"ON\"},\"socParallelAssembly\":{\"Unit\":\"1\",\"PortLabel\":\"socParallelAssembly\",\"Probing\":\"ON\"},\"vParallelAssembly\":{\"Unit\":\"V\",\"PortLabel\":\"vParallelAssembly\",\"Probing\":\"ON\"}}"
  Module4_outputs : SimscapeProbe  BoundBlock=1456  Variables="{\"batteryCurrent\":{\"Unit\":\"A\",\"PortLabel\":\"batteryCurrent\",\"Probing\":\"ON\"},\"batteryTemperature\":{\"Unit\":\"K\",\"PortLabel\":\"batteryTemperature\",\"Probing\":\"ON\"},\"batteryVoltage\":{\"Unit\":\"V\",\"PortLabel\":\"batteryVoltage\",\"Probing\":\"ON\"},\"numCycles\":{\"Unit\":\"1\",\"PortLabel\":\"numCycles\",\"Probing\":\"ON\"},\"socCell\":{\"Unit\":\"1\",\"PortLabel\":\"socCell\",\"Probing\":\"ON\"},\"socParallelAssembly\":{\"Unit\":\"1\",\"PortLabel\":\"socParallelAssembly\",\"Probing\":\"ON\"},\"vParallelAssembly\":{\"Unit\":\"V\",\"PortLabel\":\"vParallelAssembly\",\"Probing\":\"ON\"}}"
  Module5_outputs : SimscapeProbe  BoundBlock=1458  Variables="{\"batteryCurrent\":{\"Unit\":\"A\",\"PortLabel\":\"batteryCurrent\",\"Probing\":\"ON\"},\"batteryTemperature\":{\"Unit\":\"K\",\"PortLabel\":\"batteryTemperature\",\"Probing\":\"ON\"},\"batteryVoltage\":{\"Unit\":\"V\",\"PortLabel\":\"batteryVoltage\",\"Probing\":\"ON\"},\"numCycles\":{\"Unit\":\"1\",\"PortLabel\":\"numCycles\",\"Probing\":\"ON\"},\"socCell\":{\"Unit\":\"1\",\"PortLabel\":\"socCell\",\"Probing\":\"ON\"},\"socParallelAssembly\":{\"Unit\":\"1\",\"PortLabel\":\"socParallelAssembly\",\"Probing\":\"ON\"},\"vParallelAssembly\":{\"Unit\":\"V\",\"PortLabel\":\"vParallelAssembly\",\"Probing\":\"ON\"}}"
  balancingSelector1 : Selector  InputPortWidth=25  IndexOptions=Index vector (dialog)  Indices="[1  2  3  4  5]"  OutputSizes=1
  balancingSelector2 : Selector  InputPortWidth=25  IndexOptions=Index vector (dialog)  Indices="[6   7   8   9  10]"  OutputSizes=1
  balancingSelector3 : Selector  InputPortWidth=25  IndexOptions=Index vector (dialog)  Indices="[11  12  13  14  15]"  OutputSizes=1
  balancingSelector4 : Selector  InputPortWidth=25  IndexOptions=Index vector (dialog)  Indices="[16  17  18  19  20]"  OutputSizes=1
  balancingSelector5 : Selector  InputPortWidth=25  IndexOptions=Index vector (dialog)  Indices="[21  22  23  24  25]"  OutputSizes=1
  batteryCurrentMux : Mux  Inputs=5
  batteryTemperatureMux : Mux  Inputs=5
  batteryVoltageMux : Mux  Inputs=5
  numCyclesMux : Mux  Inputs=5
  socCellMux : Mux  Inputs=5
  socParallelAssemblyMux : Mux  Inputs=5
  vParallelAssemblyMux : Mux  Inputs=5
  + : PMIOPort  Side=Left
  - : PMIOPort  Port=2  Side=Right
  ClntH : PMIOPort  Port=3  Side=Right  ConnectionType=Connection: foundation.thermal.thermal
  batteryCurrent : Outport
  batteryTemperature : Outport  Port=2
  batteryVoltage : Outport  Port=3
  numCycles : Outport  Port=4
  socCell : Outport  Port=5
  socParallelAssembly : Outport  Port=6
  vParallelAssembly : Outport  Port=7
  wires:
  EVModule_outputs/1 -> [batteryCurrent1]
  batteryCurrentMux/1 -> batteryCurrent/1
  [batteryCurrent1] -> batteryCurrentMux/1
  EVModule_outputs/2 -> [batteryTemperature1]
  batteryTemperatureMux/1 -> batteryTemperature/1
  [batteryTemperature1] -> batteryTemperatureMux/1
  EVModule_outputs/3 -> [batteryVoltage1]
  batteryVoltageMux/1 -> batteryVoltage/1
  [batteryVoltage1] -> batteryVoltageMux/1
  EVModule_outputs/4 -> [numCycles1]
  numCyclesMux/1 -> numCycles/1
  [numCycles1] -> numCyclesMux/1
  EVModule_outputs/5 -> [socCell1]
  socCellMux/1 -> socCell/1
  [socCell1] -> socCellMux/1
  EVModule_outputs/6 -> [socParallelAssembly1]
  socParallelAssemblyMux/1 -> socParallelAssembly/1
  [socParallelAssembly1] -> socParallelAssemblyMux/1
  EVModule_outputs/7 -> [vParallelAssembly1]
  vParallelAssemblyMux/1 -> vParallelAssembly/1
  [vParallelAssembly1] -> vParallelAssemblyMux/1
  Module2_outputs/1 -> [batteryCurrent2]
  [batteryCurrent2] -> batteryCurrentMux/2
  Module2_outputs/2 -> [batteryTemperature2]
  [batteryTemperature2] -> batteryTemperatureMux/2
  Module2_outputs/3 -> [batteryVoltage2]
  [batteryVoltage2] -> batteryVoltageMux/2
  Module2_outputs/4 -> [numCycles2]
  [numCycles2] -> numCyclesMux/2
  Module2_outputs/5 -> [socCell2]
  [socCell2] -> socCellMux/2
  Module2_outputs/6 -> [socParallelAssembly2]
  [socParallelAssembly2] -> socParallelAssemblyMux/2
  Module2_outputs/7 -> [vParallelAssembly2]
  [vParallelAssembly2] -> vParallelAssemblyMux/2
  Module3_outputs/1 -> [batteryCurrent3]
  [batteryCurrent3] -> batteryCurrentMux/3
  Module3_outputs/2 -> [batteryTemperature3]
  [batteryTemperature3] -> batteryTemperatureMux/3
  Module3_outputs/3 -> [batteryVoltage3]
  [batteryVoltage3] -> batteryVoltageMux/3
  Module3_outputs/4 -> [numCycles3]
  [numCycles3] -> numCyclesMux/3
  Module3_outputs/5 -> [socCell3]
  [socCell3] -> socCellMux/3
  Module3_outputs/6 -> [socParallelAssembly3]
  [socParallelAssembly3] -> socParallelAssemblyMux/3
  Module3_outputs/7 -> [vParallelAssembly3]
  [vParallelAssembly3] -> vParallelAssemblyMux/3
  Module4_outputs/1 -> [batteryCurrent4]
  [batteryCurrent4] -> batteryCurrentMux/4
  Module4_outputs/2 -> [batteryTemperature4]
  [batteryTemperature4] -> batteryTemperatureMux/4
  Module4_outputs/3 -> [batteryVoltage4]
  [batteryVoltage4] -> batteryVoltageMux/4
  Module4_outputs/4 -> [numCycles4]
  [numCycles4] -> numCyclesMux/4
  Module4_outputs/5 -> [socCell4]
  [socCell4] -> socCellMux/4
  Module4_outputs/6 -> [socParallelAssembly4]
  [socParallelAssembly4] -> socParallelAssemblyMux/4
  Module4_outputs/7 -> [vParallelAssembly4]
  [vParallelAssembly4] -> vParallelAssemblyMux/4
  Module5_outputs/1 -> [batteryCurrent5]
  [batteryCurrent5] -> batteryCurrentMux/5
  Module5_outputs/2 -> [batteryTemperature5]
  [batteryTemperature5] -> batteryTemperatureMux/5
  Module5_outputs/3 -> [batteryVoltage5]
  [batteryVoltage5] -> batteryVoltageMux/5
  Module5_outputs/4 -> [numCycles5]
  [numCycles5] -> numCyclesMux/5
  Module5_outputs/5 -> [socCell5]
  [socCell5] -> socCellMux/5
  Module5_outputs/6 -> [socParallelAssembly5]
  [socParallelAssembly5] -> socParallelAssemblyMux/5
  Module5_outputs/7 -> [vParallelAssembly5]
  [vParallelAssembly5] -> vParallelAssemblyMux/5
  [balancing1] -> Converter1/1
  balancing/1 -> balancingSelector1/1, balancingSelector2/1, balancingSelector3/1, balancingSelector4/1, balancingSelector5/1
  balancingSelector1/1 -> [balancing1]
  [balancing2] -> Converter2/1
  balancingSelector2/1 -> [balancing2]
  [balancing3] -> Converter3/1
  balancingSelector3/1 -> [balancing3]
  [balancing4] -> Converter4/1
  balancingSelector4/1 -> [balancing4]
  [balancing5] -> Converter5/1
  balancingSelector5/1 -> [balancing5]
  connections:
  Module2/LConn3 -- EVModule/RConn1
  Module3/LConn3 -- Module2/RConn1
  Module4/LConn3 -- Module3/RConn1
  Module5/LConn3 -- Module4/RConn1
  EVModule/LConn3 -- +/RConn1
  Module5/RConn1 -- -/RConn1
  Converter1/RConn1 -- EVModule/LConn1
  Converter2/RConn1 -- Module2/LConn1
  Converter3/RConn1 -- Module3/LConn1
  Converter4/RConn1 -- Module4/LConn1
  Converter5/RConn1 -- Module5/LConn1
  ClntH_To_1/LConn1 -- EVModule/LConn2
  ClntH_From_1/LConn1 -- ClntH_From_2/LConn1 -- ClntH_From_3/LConn1 -- ClntH_From_4/LConn1 -- ClntH/RConn1 -- ClntH_From_5/LConn1
  ClntH_To_2/LConn1 -- Module2/LConn2
  ClntH_To_3/LConn1 -- Module3/LConn2
  ClntH_To_4/LConn1 -- Module4/LConn2
  ClntH_To_5/LConn1 -- Module5/LConn2
